simulink model "Rev14_DCtoAC_Tuning"  (R2018a)
settings: Solver=VariableStepAuto  StartTime=0.0  StopTime=5  MaxStep=1e-4  RelTol=1e-3  EnableMultiTasking=on
values from neighbouring files (symbols this model uses):
  bw = 4 * 2 *pi    (= 25.1327412287)    [modelCfg.m]
  C = 50e-3    (= 0.05)    [modelCfg.m]
  CinpFtr = 1e-9    (= 1e-09)    [modelCfg.m]
  f = 50    [controlhinf.m]    (also in controlhinf2.m; modelCfg.m; psd_score.m = (1/avgT_samp)/n*(0:floor((n-1)/2)))
  floorcoeff = 10^(floor_dB/10+ 8/10)*bw    (= 1.58576876652e-06)    [modelCfg.m]
  Idcmax = Pmax / Vdc    (= 24.2857142857)    [modelCfg.m]
  Ki_i = R./tau .* ICtrl_coeff(2)    [modelCfg.m]
  Ki_v = VCtrlTune(4) .* -1 .* (Kp_v .^ 2)/ (4.*C)    [modelCfg.m]
  Kp_i = L./tau .* ICtrl_coeff(1)    [modelCfg.m]
  Kp_v = VCtrlTune(3) .* -2 .* maxDeltaIdc ./ (exp(1) .* maxDeltaVdc)    [modelCfg.m]
  Kr_i1 = Ki_i .* ICtrl_coeff(3)    [modelCfg.m]
  Kr_i2 = Ki_i .* ICtrl_coeff(4)    [modelCfg.m]
  Kr_i3 = Ki_i .* ICtrl_coeff(5)    [modelCfg.m]
  Kr_i4 = Ki_i .* ICtrl_coeff(6)    [modelCfg.m]
  L = 570e-6    (= 0.00057)    [controlhinf.m]    (also in controlhinf2.m; modelCfg.m)
  R = 3e-3    (= 0.003)    [controlhinf.m]    (also in controlhinf2.m = 0.03; modelCfg.m)
  RinpFtr = 15e3    (= 15000)    [modelCfg.m]
  tau = 2e-3    (= 0.002)    [modelCfg.m]
  Vac = 40    [modelCfg.m]
  Vacpp = Vac .* sqrt(2)    [modelCfg.m]
  Vdc = 70    [modelCfg.m]
  w_e = 2*pi*f    (= 314.159265359)    [modelCfg.m]
  w_n = 2 * w_e    (= 628.318530718)    [modelCfg.m]
undefined symbols (not defined in the file or in its folder): sigbuilder_block
libraries: powerlib x14, discretizing x12, simulink x4, dspstat3 x1, powerlib_meascontrol x1
settings Model: Creator=cmp14  LastModifiedBy=Chung
settings SolverCC: ZeroCrossAlgorithm=Adaptive
settings DataIOCC: OutputSaveName=simStabilityNew
settings DebuggingCC: IgnoredZcDiagnostic=none
settings ModelReferenceCC: ParallelModelReferenceMATLABWorkerInit=Load Top Model
settings CodeAppCC: StateflowObjectComments=on
settings SimscapeCC: SimscapeNormalizeSystem=off

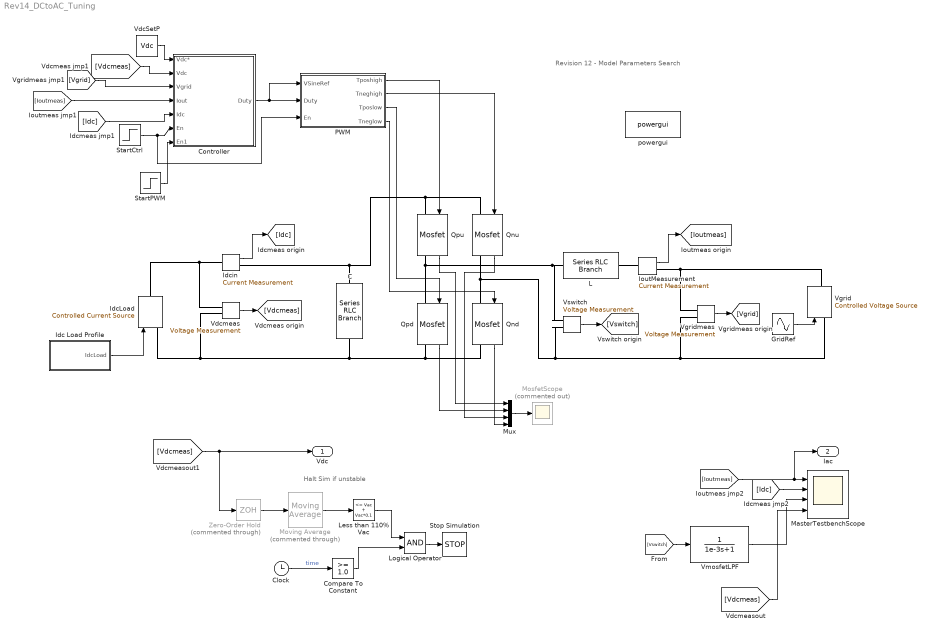
== system Rev14_DCtoAC_Tuning ==
  note: Halt Sim if unstable
  note: Revision 12 - Model Parameters Search
  C : powerlib/Elements/Series RLC Branch  LConnTagsString=__new0  RConnTagsString=__new0  BranchType=RC  Resistance=R  Inductance=1e-3  SetiL0=off  InitialCurrent=0  Capacitance=C  Setx0=on  InitialVoltage=Vdc  Measurements=None
  Clock : Clock
      settings: Decimation=1000
  Compare To Constant : simulink/Logic and Bit Operations/Compare To Constant  relop=>=  const=1.0  OutDataTypeStr=boolean
  Controller : Subsystem
  GridRef : Sin  Amplitude=Vacpp  Frequency=2*pi*f  Phase=pi  SampleTime=0
  Idc Load Profile : Subsystem  Tag=STV Subsys  LoadFcn=sigbuilder_block('load');  StartFcn=sigbuilder_block('start');  StopFcn=sigbuilder_block('stop');  ClipboardFcn=sigbuilder_block('clipboard');  mask(Sigbuilder block){tuvar=[0:10]}
      mask help: Simulink:masks:SigbuilderBlock_MD
      mask init:
      | if ~strcmp(get_param(bdroot(gcbh),'SimulationStatus'),'stopped') tuvar = sigbuilder_block('maskInit'); end
      settings: CopyFcn=sigbuilder_block('copy');  DeleteFcn=sigbuilder_block('delete');  ModelCloseFcn=sigbuilder_block('modelClose');  PreSaveFcn=sigbuilder_block('preSave');  PauseFcn=sigbuilder_block('pause');  ContinueFcn=sigbuilder_block('continue');  NameChangeFcn=sigbuilder_block('namechange');  OpenFcn=sigbuilder_block('open',[6 30 1012.5 447.75 ]);  CloseFcn=sigbuilder_block('close');
      mask Display: plot(0, 0, 100, 100,[2, 2, 32, 32, 2], [68, 8, 8, 68, 68],[32, 2], [38, 38], [32, 19, 2],[53, 60, 44], [32, 17, 17, 2],[16, 16, 31, 31]);txt = getActiveGroup(gcbh);text(2, 100, txt,'verticalAlignment', 'top');
  IdcLoad : powerlib/Electrical Sources/Controlled Current Source  Initialize=on  Source_Type=AC  Amplitude=0  Phase=0  Frequency=0  Measurements=None
  Idcin : powerlib/Measurements/Current Measurement  PhasorSimulation=off  OutputType=Complex  PSBequivalent=0
  IoutMeasurement : powerlib/Measurements/Current Measurement  PhasorSimulation=off  OutputType=Complex  PSBequivalent=0
  L : powerlib/Elements/Series RLC Branch  LConnTagsString=__new0  RConnTagsString=__new0  BranchType=RL  Resistance=R  Inductance=L  SetiL0=off  InitialCurrent=0  Capacitance=1e-6  Setx0=off  InitialVoltage=0  Measurements=None
  Less than 110% Vac : simulink/Logic and Bit Operations/Compare To Constant  relop=<=  const=Vac + Vac*0.1  OutDataTypeStr=boolean
  Logical Operator : Logic  AllPortsSameDT=off  OutDataTypeStr=boolean
  MasterTestbenchScope : Scope  NumInputPorts=4
  MosfetScope : Scope  Commented=on
  Moving Average : dspstat3/Moving Average  Commented=through  Method=Sliding window  ForgettingFactorPort=off  SpecifyWindowLength=on  WindowLength=1000  ForgettingFactor=0.9  SimulateUsing=Code generation
  Mux : Mux
  PWM : Subsystem
  Qnd : powerlib/Power Electronics/Mosfet  Ron=65e-3  Lon=0  Rd=0.01  Vfd=1  IC=0  Rs=1e5  Cs=inf  Measurements=on
  Qnu : powerlib/Power Electronics/Mosfet  Ron=65e-3  Lon=0  Rd=0.01  Vfd=1  IC=0  Rs=1e5  Cs=inf  Measurements=on
  Qpd : powerlib/Power Electronics/Mosfet  Ron=65e-3  Lon=0  Rd=0.01  Vfd=1  IC=0  Rs=1e5  Cs=inf  Measurements=on
  Qpu : powerlib/Power Electronics/Mosfet  Ron=65e-3  Lon=0  Rd=0.01  Vfd=1  IC=0  Rs=1e5  Cs=inf  Measurements=on
  StartCtrl : Step  Time=0.2  SampleTime=0
  StartPWM : Step  Time=0.21  SampleTime=0
  Stop Simulation : Stop
  VdcSetP : Constant  Value=Vdc
  Vdcmeas : powerlib/Measurements/Voltage Measurement  PhasorSimulation=off  OutputType=Complex  PSBequivalent=0
  Vgrid : powerlib/Electrical Sources/Controlled Voltage Source  Initialize=on  Source_Type=AC  Amplitude=Vacpp  Phase=0  Frequency=f  Measurements=None
  Vgridmeas : powerlib/Measurements/Voltage Measurement  PhasorSimulation=off  OutputType=Complex  PSBequivalent=0
  VmosfetLPF : TransferFcn  Denominator=[1e-3 1]
  Vswitch : powerlib/Measurements/Voltage Measurement  PhasorSimulation=off  OutputType=Complex  PSBequivalent=0
  Zero-Order Hold : ZeroOrderHold  Commented=through  SampleTime=-1
  powergui : powerlib/powergui  Priority=1  SimulationMode=Continuous  SampleTime=50e-6  frequency=60  Iterations=50  frequencyindice=0  Pbase=100e6  ErrMax=1e-4  UnitsV=kV  UnitsW=MW  buscounter=0  FunctionMessages=off  echomessages=off  EnableUseOfTLC=off  CurrentSourceSwitches=off  DisableSnubberDevices=off  DisableRonSwitches=off  DisableVfSwitches=off  DisplayEquations=off  SolverType=Tustin/Backward Euler (TBE)  Interpol=off  ExternalGateDelay=off  methode=off  Ts=100  x0status=blocks  SPID=on  SwTol=0  HookPort=off  RestoreLinks=warning  ResistiveCurrentMeasurement=off  Frange=[0:2:500]  Ylog=off  Xlog=on  ShowGrid=off  save=off  variable=ZData  structure=0  ZoomFFT=off  StartTime=0.0  cycles=1  DisplayStyle=1  fundamental=60  FreqAxis=off  MaxFrequency=1000  frequencyindicesteady=1  RmsSteady=1  display=off
  Vdc : Outport
  Iac : Outport  Port=2
  wires:
  VdcSetP/1 -> Controller/1(Vdc*)
  Vdcmeas/1 -> [Vdcmeas]
  PWM/4(Tneglow) -> Qnd/1
  PWM/3(Tposlow) -> Qpd/1
  PWM/1(Tposhigh) -> Qpu/1
  PWM/2(Tneghigh) -> Qnu/1
  [Vdcmeas] -> MasterTestbenchScope/4
  Idc Load Profile/1(IdcLoad) -> IdcLoad/1
  VmosfetLPF/1 -> MasterTestbenchScope/3
  GridRef/1 -> Vgrid/1
  [Vdcmeas] -> Controller/2(Vdc)
  [Vgrid] -> Controller/3(Vgrid)
  [Ioutmeas] -> Controller/4(Iout)
  Vswitch/1 -> [Vswitch]
  Controller/1(Duty) -> PWM/1(VSineRef), PWM/2(Duty)
  [Vswitch] -> VmosfetLPF/1
  [Ioutmeas] -> Iac/1, MasterTestbenchScope/1
  Idcin/1 -> [Idc]
  [Idc] -> Controller/5(Idc)
  Vgridmeas/1 -> [Vgrid]
  IoutMeasurement/1 -> [Ioutmeas]
  [Vdcmeas] -> Zero-Order Hold/1, Vdc/1
  [Idc] -> MasterTestbenchScope/2
  Qpu/1 -> Mux/1
  Qpd/1 -> Mux/2
  Qnu/1 -> Mux/3
  Qnd/1 -> Mux/4
  Mux/1 -> MosfetScope/1
  Zero-Order Hold/1 -> Moving Average/1
  Moving Average/1 -> Less than 110% Vac/1
  Clock/1 -> Compare To Constant/1  "time"
  Compare To Constant/1 -> Logical Operator/2
  Less than 110% Vac/1 -> Logical Operator/1
  Logical Operator/1 -> Stop Simulation/1
  StartCtrl/1 -> PWM/3(En), Controller/6(En)
  StartPWM/1 -> Controller/7(En1)
  connections:
  IoutMeasurement/LConn1 -- L/RConn1
  Vswitch/LConn1 -- L/LConn1 -- Qpd/LConn1 -- Qpu/RConn1
  Qpd/RConn1 -- Qnd/RConn1 -- IdcLoad/LConn1 -- Vdcmeas/LConn2 -- C/RConn1
  Qpu/LConn1 -- Idcin/RConn1 -- C/LConn1 -- Qnu/LConn1
  Qnu/RConn1 -- Qnd/LConn1 -- Vgrid/LConn1 -- Vgridmeas/LConn2 -- Vswitch/LConn2
  IoutMeasurement/RConn1 -- Vgridmeas/LConn1 -- Vgrid/RConn1
  Vdcmeas/LConn1 -- IdcLoad/RConn1 -- Idcin/LConn1

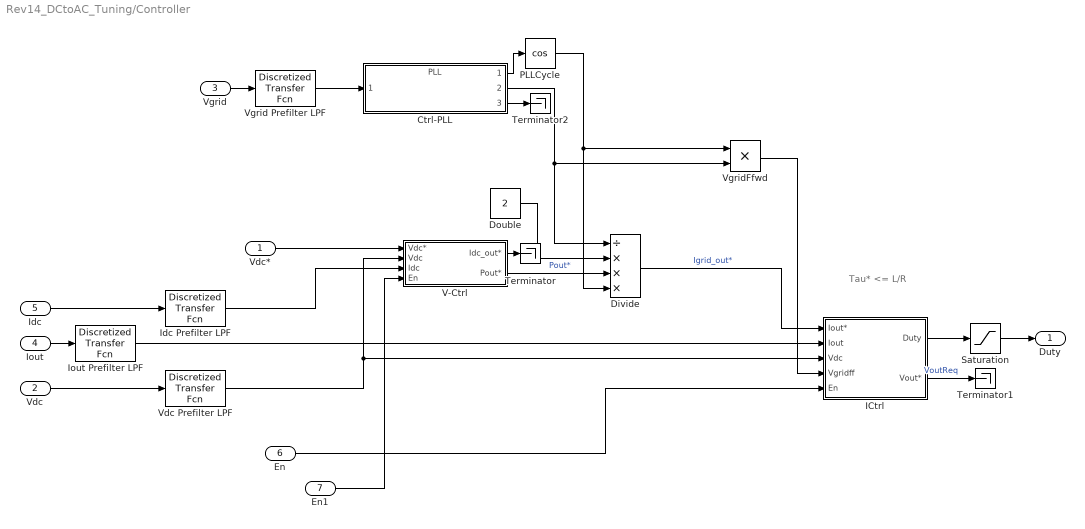
== system Rev14_DCtoAC_Tuning/Controller ==
  note: Tau* <= L/R
  Vdc* : Inport
  Vdc : Inport  Port=2
  Vgrid : Inport  Port=3
  Iout : Inport  Port=4
  Idc : Inport  Port=5
  En : Inport  Port=6
  En1 : Inport  Port=7
  Ctrl-PLL : ModelReference  ModelNameDialog=PLL.slx  SimulationMode=Normal  ModelReferenceVersion=1.11
  Divide : Product  Inputs=/***
  Double : Constant  Value=2
  ICtrl : Subsystem  TreatAsAtomicUnit=on
  Idc Prefilter LPF : discretizing/Discretized Transfer Fcn  Numerator=[1]  Denominator=[RinpFtr*CinpFtr 1]  AbsTol=auto  SampleTime=5.0e-5  method=tustin  Wc=1
  Iout Prefilter LPF : discretizing/Discretized Transfer Fcn  Numerator=[1]  Denominator=[RinpFtr*CinpFtr 1]  AbsTol=auto  SampleTime=5.0e-5  method=tustin  Wc=1
  PLLCycle : Trigonometry  Operator=cos
  Saturation : Saturate  UpperLimit=1  LowerLimit=-1  LinearizeAsGain=off
  Terminator : Terminator
  Terminator1 : Terminator
  Terminator2 : Terminator
  V-Ctrl : Subsystem  TreatAsAtomicUnit=on
  Vdc Prefilter LPF : discretizing/Discretized Transfer Fcn  Numerator=[1]  Denominator=[RinpFtr*CinpFtr 1]  AbsTol=auto  SampleTime=5.0e-5  method=tustin  Wc=1
  Vgrid Prefilter LPF : discretizing/Discretized Transfer Fcn  Numerator=[1]  Denominator=[RinpFtr*CinpFtr 1]  AbsTol=auto  SampleTime=5.0e-5  method=tustin  Wc=1
  VgridFfwd : Product  Inputs=**
  Duty : Outport
  wires:
  Iout/1 -> Iout Prefilter LPF/1
  Divide/1 -> ICtrl/1(Iout*)  "Igrid_out*"
  Vdc*/1 -> V-Ctrl/1(Vdc*)
  Vgrid/1 -> Vgrid Prefilter LPF/1
  Vdc/1 -> Vdc Prefilter LPF/1
  V-Ctrl/2(Pout*) -> Divide/3  "Pout*"
  ICtrl/1(Duty) -> Saturation/1
  Saturation/1 -> Duty/1
  En/1 -> ICtrl/5(En)
  Double/1 -> Divide/2
  Ctrl-PLL/1 -> PLLCycle/1
  Idc/1 -> Idc Prefilter LPF/1
  V-Ctrl/1(Idc_out*) -> Terminator/1
  PLLCycle/1 -> Divide/4, VgridFfwd/1
  VgridFfwd/1 -> ICtrl/4(Vgridff)
  Ctrl-PLL/2 -> Divide/1, VgridFfwd/2
  ICtrl/2(Vout*) -> Terminator1/1  "VoutReq"
  Ctrl-PLL/3 -> Terminator2/1
  En1/1 -> V-Ctrl/4(En)
  Idc Prefilter LPF/1 -> V-Ctrl/3(Idc)
  Vdc Prefilter LPF/1 -> ICtrl/3(Vdc), V-Ctrl/2(Vdc)
  Vgrid Prefilter LPF/1 -> Ctrl-PLL/1
  Iout Prefilter LPF/1 -> ICtrl/2(Iout)

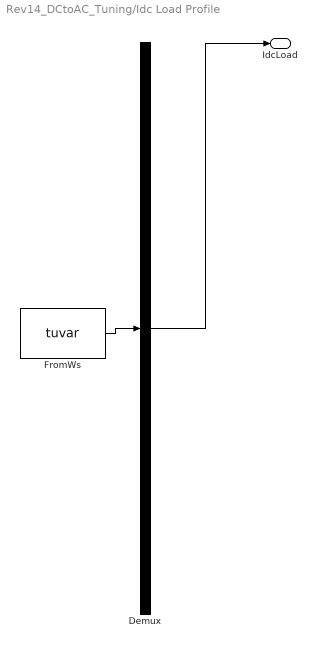
== system Rev14_DCtoAC_Tuning/Idc Load Profile ==
  Demux : Demux  Tag=STV Demux  Outputs=1
  FromWs : FromWorkspace  Tag=STV FromWs  VariableName=tuvar  SampleTime=0
      SigBuilderData=|
      | common.afterFinalStr = 'Extrapolate'
      | common.sampleTime = 0
      | dataSet.timeRange = [0 10]
      | dataSet.name = 'Group 1'
      | sbobj.Groups.Name = 'Group 1'
      | sbobj.Groups.Signals.Name = 'IdcLoad'
      | sbobj.Groups.Signals.XData = [0 0.5 0.5 1.01 1.01 1.49 1.49 2 2 2.48 2.48 2.99 2.99 3.99 3.99 4.56 4.56 10]
      | sbobj.Groups.Signals.YData = [0.1 0 16 16 0.1 0.1 -23.9 -23.9 0.1 0.1 20.1 20.2 -16.8 -17 24.1 24.2 0.1 0.1]
  IdcLoad : Outport  Tag=STV Outport
  wires:
  Demux/1 -> IdcLoad/1
  FromWs/1 -> Demux/1

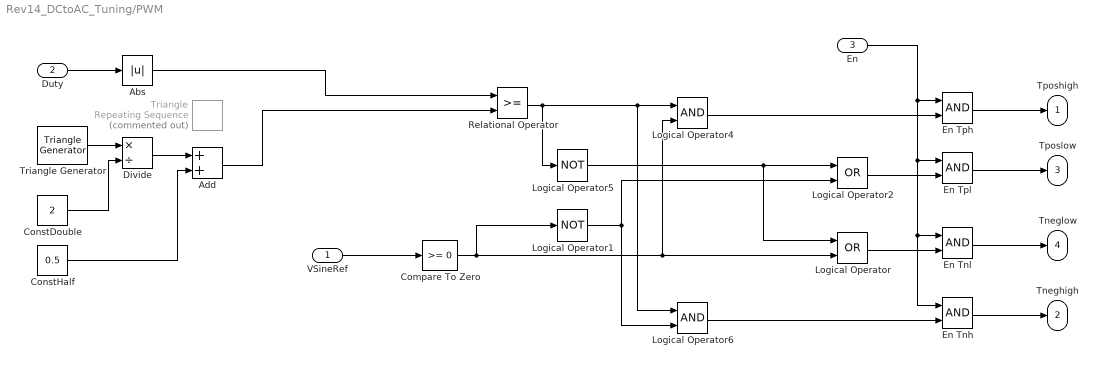
== system Rev14_DCtoAC_Tuning/PWM ==
  VSineRef : Inport
  Duty : Inport  Port=2
  En : Inport  Port=3
  Abs : Abs
  Add : Sum
  Compare To Zero : simulink/Logic and Bit Operations/Compare To Zero  relop=>=  OutDataTypeStr=boolean
  ConstDouble : Constant  Value=2
  ConstHalf : Constant  Value=0.5
  Divide : Product  Inputs=*/
  En Tnh : Logic  AllPortsSameDT=off  OutDataTypeStr=boolean
  En Tnl : Logic  AllPortsSameDT=off  OutDataTypeStr=boolean
  En Tph : Logic  AllPortsSameDT=off  OutDataTypeStr=boolean
  En Tpl : Logic  AllPortsSameDT=off  OutDataTypeStr=boolean
  Logical Operator : Logic  Operator=OR  AllPortsSameDT=off  OutDataTypeStr=boolean
  Logical Operator1 : Logic  Operator=NOT  AllPortsSameDT=off  OutDataTypeStr=boolean
  Logical Operator2 : Logic  Operator=OR  AllPortsSameDT=off  OutDataTypeStr=boolean
  Logical Operator4 : Logic  AllPortsSameDT=off  OutDataTypeStr=boolean
  Logical Operator5 : Logic  Operator=NOT  AllPortsSameDT=off  OutDataTypeStr=boolean
  Logical Operator6 : Logic  AllPortsSameDT=off  OutDataTypeStr=boolean
  Relational Operator : RelationalOperator  OutDataTypeStr=boolean  RndMeth=Nearest
  Triangle : simulink/Sources/Repeating Sequence  Commented=on  rep_seq_t=[0 5e-5]  rep_seq_y=[0 1]
  Triangle Generator : powerlib_meascontrol/Pulse & Signal Generators/Triangle Generator  Freq=f_s  Phase=90  Ts=0
  Tposhigh : Outport
  Tneghigh : Outport  Port=2
  Tposlow : Outport  Port=3
  Tneglow : Outport  Port=4
  wires:
  VSineRef/1 -> Compare To Zero/1
  Compare To Zero/1 -> Logical Operator1/1, Logical Operator4/2, Logical Operator/2
  Logical Operator5/1 -> Logical Operator/1, Logical Operator2/1
  Relational Operator/1 -> Logical Operator5/1, Logical Operator6/1, Logical Operator4/1
  Logical Operator1/1 -> Logical Operator6/2, Logical Operator2/2
  Triangle Generator/1 -> Divide/1
  Divide/1 -> Add/1
  ConstDouble/1 -> Divide/2
  ConstHalf/1 -> Add/2
  Duty/1 -> Abs/1
  Add/1 -> Relational Operator/2
  Abs/1 -> Relational Operator/1
  En/1 -> En Tnh/1, En Tnl/1, En Tpl/1, En Tph/1
  En Tnh/1 -> Tneghigh/1
  En Tnl/1 -> Tneglow/1
  En Tpl/1 -> Tposlow/1
  En Tph/1 -> Tposhigh/1
  Logical Operator4/1 -> En Tph/2
  Logical Operator6/1 -> En Tnh/2
  Logical Operator/1 -> En Tnl/2
  Logical Operator2/1 -> En Tpl/2

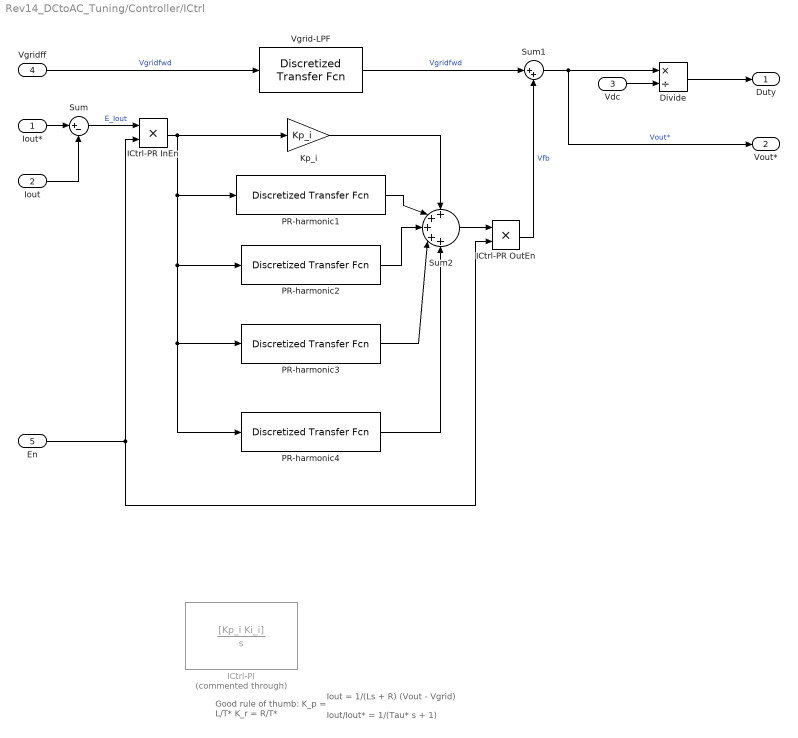
== system Rev14_DCtoAC_Tuning/Controller/ICtrl ==
  note: Iout/Iout* = 1/(Tau* s + 1)
  note: Iout = 1/(Ls + R) (Vout - Vgrid)
  note: Good rule of thumb:
      | K_p = L/T*
      | K_r = R/T*
  Iout* : Inport
  Iout : Inport  Port=2
  Vdc : Inport  Port=3
  Vgridff : Inport  Port=4
  En : Inport  Port=5
  Divide : Product  Inputs=*/
  ICtrl-PI : TransferFcn  Commented=through  Numerator=[Kp_i Ki_i]  Denominator=[1 0]
  ICtrl-PR InEn : Product
  ICtrl-PR OutEn : Product
  Kp_i : Gain  Gain=Kp_i
  PR-harmonic1 : discretizing/Discretized Transfer Fcn  Numerator=[Kr_i1 0]  Denominator=[1 0 (2*pi*f)^2]  AbsTol=auto  SampleTime=5.0e-5  method=tustin  Wc=1
  PR-harmonic2 : discretizing/Discretized Transfer Fcn  Numerator=[Kr_i2 0]  Denominator=[1 0 (2*pi*f*3)^2]  AbsTol=auto  SampleTime=5.0e-5  method=tustin  Wc=1
  PR-harmonic3 : discretizing/Discretized Transfer Fcn  Numerator=[Kr_i3 0]  Denominator=[1 0 (2*pi*f*5)^2]  AbsTol=auto  SampleTime=5.0e-5  method=tustin  Wc=1
  PR-harmonic4 : discretizing/Discretized Transfer Fcn  Numerator=[Kr_i4 0]  Denominator=[1 0 (2*pi*f*7)^2]  AbsTol=auto  SampleTime=5.0e-5  method=tustin  Wc=1
  Sum : Sum  Inputs=|+-
  Sum1 : Sum  Inputs=|++
  Sum2 : Sum  Inputs=+++++
  Vgrid-LPF : discretizing/Discretized Transfer Fcn  Numerator=[1]  Denominator=[tau 1]  AbsTol=auto  SampleTime=5.0e-5  method=tustin  Wc=1
  Duty : Outport
  Vout* : Outport  Port=2
  wires:
  Sum1/1 -> Vout*/1, Divide/1  "Vout*"
  Iout*/1 -> Sum/1
  Iout/1 -> Sum/2
  Vdc/1 -> Divide/2
  Sum/1 -> ICtrl-PR InEn/1  "E_Iout"
  Divide/1 -> Duty/1
  En/1 -> ICtrl-PR InEn/2, ICtrl-PR OutEn/2
  Kp_i/1 -> Sum2/1
  Sum2/1 -> ICtrl-PR OutEn/1
  PR-harmonic1/1 -> Sum2/2
  PR-harmonic2/1 -> Sum2/3
  ICtrl-PR OutEn/1 -> Sum1/2  "Vfb"
  Vgridff/1 -> Vgrid-LPF/1  "Vgridfwd"
  PR-harmonic3/1 -> Sum2/4
  PR-harmonic4/1 -> Sum2/5
  ICtrl-PR InEn/1 -> PR-harmonic1/1, PR-harmonic4/1, PR-harmonic3/1, PR-harmonic2/1, Kp_i/1
  Vgrid-LPF/1 -> Sum1/1  "Vgridfwd"

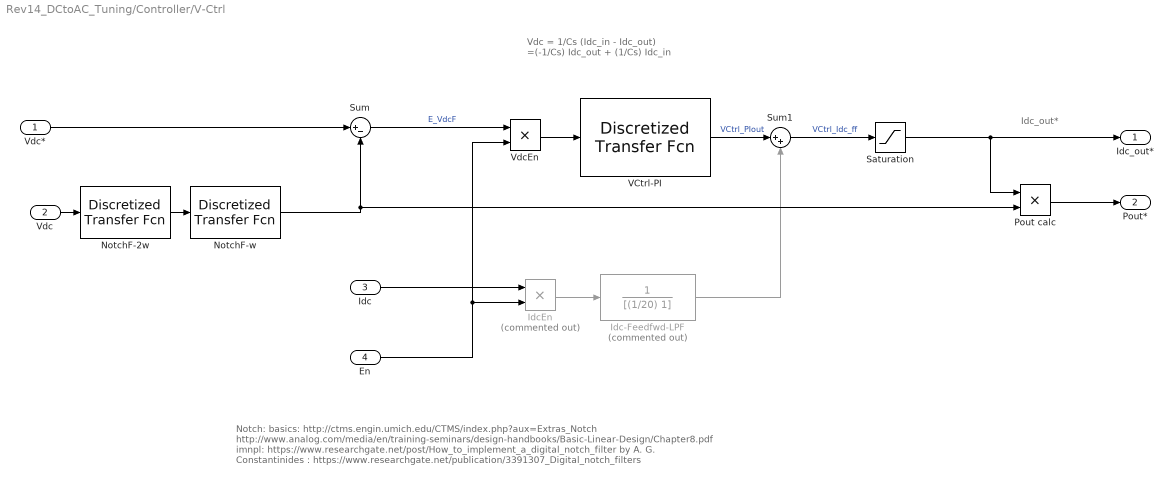
== system Rev14_DCtoAC_Tuning/Controller/V-Ctrl ==
  note: Notch:
      | basics: http://ctms.engin.umich.edu/CTMS/index.php?aux=Extras_Notch
      | http://www.analog.com/media/en/training-seminars/design-handbooks/Basic-Linear-Design/Chapter8.pdf
      | imnpl: https://www.researchgate.net/post/How_to_implement_a_digital_notch_filter by
      | A. G. Constantinides : https://www.researchgate.net/publication/3391307_Digital_notch_filters
  note: Idc_out*
  note: Vdc = 1/Cs (Idc_in - Idc_out)
      | =(-1/Cs) Idc_out + (1/Cs) Idc_in
  Vdc* : Inport
  Vdc : Inport  Port=2
  Idc : Inport  Port=3
  En : Inport  Port=4
  Idc-Feedfwd-LPF : TransferFcn  Commented=on  Denominator=[(1/20) 1]
  IdcEn : Product  Commented=on
  NotchF-2w : discretizing/Discretized Transfer Fcn  Numerator=[1 floorcoeff (w_n^2)]  Denominator=[1 2*bw w_n^2]  AbsTol=auto  SampleTime=5.0e-5  method=tustin  Wc=1
  NotchF-w : discretizing/Discretized Transfer Fcn  Numerator=[1 floorcoeff (w_e^2)]  Denominator=[1 2*bw w_e^2]  AbsTol=auto  SampleTime=5.0e-5  method=tustin  Wc=1
  Pout calc : Product  Inputs=**
  Saturation : Saturate  UpperLimit=2*Idcmax  LowerLimit=-2*Idcmax  LinearizeAsGain=off
  Sum : Sum  Inputs=|+-
  Sum1 : Sum  Inputs=|++
  VCtrl-PI : discretizing/Discretized Transfer Fcn  Numerator=[Kp_v Ki_v]  Denominator=[1 0]  AbsTol=auto  SampleTime=5.0e-5  method=tustin  Wc=1
  VdcEn : Product
  Idc_out* : Outport
  Pout* : Outport  Port=2
  wires:
  Pout calc/1 -> Pout*/1
  Vdc*/1 -> Sum/1
  En/1 -> IdcEn/2, VdcEn/2
  VdcEn/1 -> VCtrl-PI/1
  Idc/1 -> IdcEn/1
  IdcEn/1 -> Idc-Feedfwd-LPF/1
  VCtrl-PI/1 -> Sum1/1  "VCtrl_PIout"
  Idc-Feedfwd-LPF/1 -> Sum1/2
  Saturation/1 -> Idc_out*/1, Pout calc/1
  Sum1/1 -> Saturation/1  "VCtrl_Idc_ff"
  Sum/1 -> VdcEn/1  "E_VdcF"
  NotchF-w/1 -> Sum/2, Pout calc/2
  NotchF-2w/1 -> NotchF-w/1
  Vdc/1 -> NotchF-2w/1
